simulink model "slcpia"  (R2016a)
settings: Solver=ode45  SolverMode=SingleTasking  StartTime=0.0  StopTime=250  RelTol=1e-3
PreLoadFcn:
  | initcp
libraries: fuzblock x1
CloseFcn:
  | AnimFigTitle = [winName, ': Cart & Pole Animation']; AnimFigH = findobj(0,'Name',AnimFigTitle); close(AnimFigH)
settings Model: FPTRunName=Active  Creator=The MathWorks, Inc.  LastModifiedBy=as16542
settings DataIOCC: LimitDataPoints=on  SaveFormat=Array
settings OptimizationCC: BlockReduction=off  BooleanDataType=off
settings DebuggingCC: SaveWithParameterizedLinksMsg=none  UnderspecifiedInitializationDetection=Classic  MergeDetectMultiDrivingBlocksExec=none  SignalResolutionControl=TryResolveAllWithWarning
settings HardwareCC: ProdBitPerPointer=32  ProdLargestAtomicFloat=None  ProdIntDivRoundTo=Undefined  ProdEndianess=Unspecified  ProdWordSize=32  ProdHWDeviceType=32-bit Generic  TargetUnknown=on
settings ModelReferenceCC: PropagateSignalLabelsOutOfModel=off
settings ConfigComp: CovModelRefEnable=Off  CovSFcnEnable=off

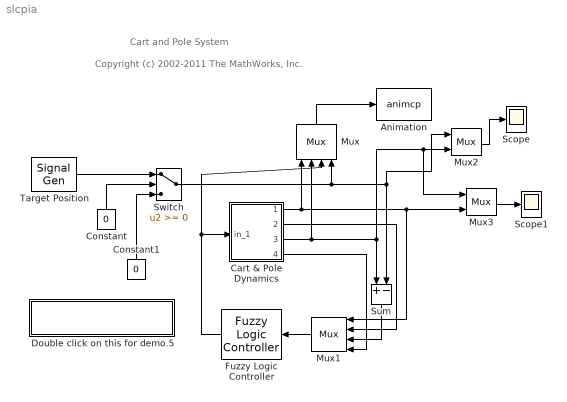
== system slcpia ==
  note: Copyright (c) 2002-2011 The MathWorks, Inc.
  note: Cart and Pole System
  Animation : S-Function  FunctionName=animcp  SFunctionDeploymentMode=off  EnableBusSupport=off
  Cart & Pole Dynamics : Subsystem  mask(Cart & Pole){init_cond=[0, 0, 2, 0], specs=[1.0, 0.1, 1.0, 9.8]}
      mask prompts: init_cond "Initial Conditions (angle, angular velocity, cart position and cart velocity):"; specs "Physical Specifications (pole length, pole mass, cart mass and g):"
      mask help: Inverted Pendulum (cart & pole)
      mask init:
      | l=specs(1)/2;m=specs(2);mc=specs(3);g=specs(4);
      mask Help: Inverted Pendulum
      mask Display: plot(-4,-1,4,6,[0 3 2.8 -0.2 0],[1 5 5.15 1.15 1],[-1 -1 1 1 -1],[1 0 0 1 1],[-3.5 3.5],[0 0])
  Constant : Constant  Value=0
  Constant1 : Constant  Value=0
  Double click on this for demo.5 : Subsystem
      settings: OpenFcn=initcp
      mask Display: disp('Variable Initialization')
  Fuzzy Logic Controller : fuzblock/Fuzzy Logic  Controller  fis=main_fis
  Mux : Mux
  Mux1 : Mux
  Mux2 : Mux  Inputs=2
  Mux3 : Mux  Inputs=2
  Scope : Scope
  Scope1 : Scope
  Sum : Sum  Inputs=+-  SaturateOnIntegerOverflow=on  InputSameDT=on  OutDataTypeStr=Inherit: Same as first input
  Switch : Switch  SaturateOnIntegerOverflow=on  InputSameDT=on
  Target Position : SignalGenerator  Amplitude=1.500000  Frequency=0.128320  Units=rad/sec
  wires:
  Target Position/1 -> Switch/1
  Constant/1 -> Switch/2
  Mux2/1 -> Scope/1
  Mux/1 -> Animation/1
  Cart & Pole Dynamics/4(out_4) -> Mux1/4
  Switch/1 -> Mux2/1, Sum/2, Mux/4
  Fuzzy Logic Controller/1 -> Mux/3, Cart & Pole Dynamics/1(in_1)
  Cart & Pole Dynamics/3(out_3) -> Mux3/1, Mux2/2, Sum/1, Mux/2
  Cart & Pole Dynamics/1(out_1) -> Mux/1, Mux1/1, Mux3/2
  Cart & Pole Dynamics/2(out_2) -> Mux1/2
  Sum/1 -> Mux1/3
  Mux1/1 -> Fuzzy Logic Controller/1
  Mux3/1 -> Scope1/1
  Constant1/1 -> Switch/3

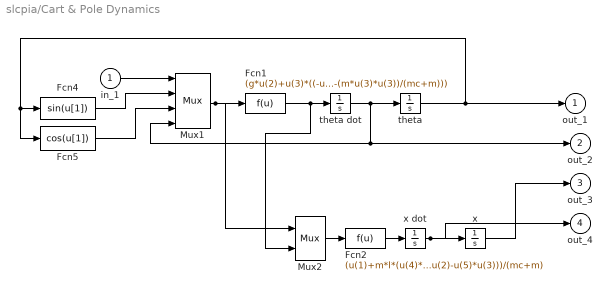
== system slcpia/Cart & Pole Dynamics ==
  in_1 : Inport
  Fcn1 : Fcn  Expr=(g*u(2)+u(3)*((-u(1)-m*l*u(4)*u(4)*u(2))/(mc+m)))/(l*(4/3-(m*u(3)*u(3))/(mc+m)))
  Fcn2 : Fcn  Expr=(u(1)+m*l*(u(4)*u(4)*u(2)-u(5)*u(3)))/(mc+m)
  Fcn4 : Fcn
  Fcn5 : Fcn  Expr=cos(u[1])
  Mux1 : Mux
  Mux2 : Mux  Inputs=[4,1]
  theta : Integrator  InitialCondition=init_cond(1)
  theta dot : Integrator  InitialCondition=init_cond(2)
  x : Integrator  InitialCondition=init_cond(3)
  x dot : Integrator  InitialCondition=init_cond(4)
  out_1 : Outport  InitialOutput=0
  out_2 : Outport  Port=2  InitialOutput=0
  out_3 : Outport  Port=3  InitialOutput=0
  out_4 : Outport  Port=4  InitialOutput=0
  wires:
  in_1/1 -> Mux1/1
  x/1 -> out_3/1
  x dot/1 -> out_4/1, x/1
  Mux1/1 -> Fcn1/1, Mux2/1
  Mux2/1 -> Fcn2/1
  Fcn2/1 -> x dot/1
  Fcn1/1 -> Mux2/2, theta dot/1
  theta dot/1 -> Mux1/4, out_2/1, theta/1
  Fcn4/1 -> Mux1/2
  Fcn5/1 -> Mux1/3
  theta/1 -> Fcn4/1, Fcn5/1, out_1/1

== system slcpia/Double click on this for demo.5 ==
